simulink model "Solar_Panel_Mathematical_Modelling"  (R2020a)
settings: Solver=VariableStepAuto  StartTime=0.0  StopTime=10.0  RelTol=1e-3
values from neighbouring files (symbols this model uses):
  K = numerator ./ denominator    [Finding_maxima_and_minima_of_any_function.m]    (also in Full_bridge_LLC_resonant_tank_gain_graphs.m; Series_LLC_resonant_converter_calculations.m; Series_LLC_resonant_converter_calculations_2.m; resonant_tank_gain.m)
  Ki = 0.2    [PID_Controller.m]
  n = 1    [Converter_Magnetics_calculations.m]    (also in Series_LLC_resonant_converter_calculations_3.m = 0.0133333333333)
  Ns = 100    [Full_bridge_LLC_resonant_tank_gain_graphs.m]    (also in Series_LLC_resonant_converter_calculations.m; Series_LLC_resonant_converter_calculations_2.m = 75; Series_LLC_resonant_converter_calculations_3.m = 75)
undefined symbols (not defined in the file or in its folder): Eg0, Isc, N, q, Rs, Rsh, Tn, Voc
libraries: simulink x1
settings Model: Creator=HP  LastModifiedBy=HP

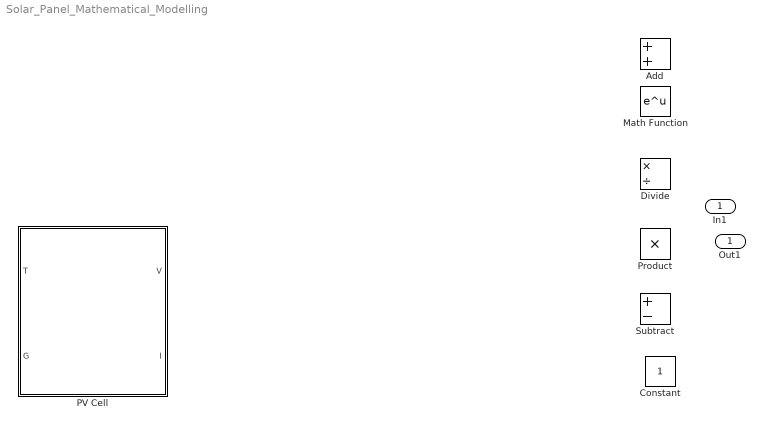
== system Solar_Panel_Mathematical_Modelling ==
  In1 : Inport
  Add : Sum
  Constant : Constant
  Divide : Product  Inputs=*/
  Math Function : Math  SaturateOnIntegerOverflow=on
  PV Cell : Subsystem
  Product : Product
  Subtract : Sum  Inputs=+-
  Out1 : Outport

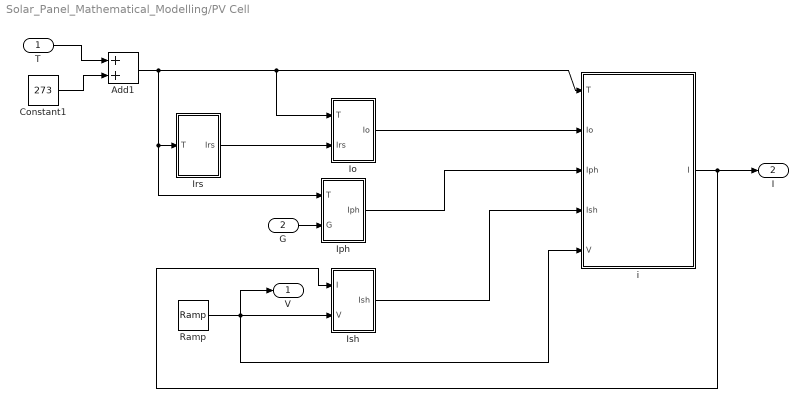
== system Solar_Panel_Mathematical_Modelling/PV Cell ==
  T : Inport
  G : Inport  Port=2
  Add1 : Sum
  Constant1 : Constant  Value=273
  Io : Subsystem
  Iph : Subsystem
  Irs : Subsystem
  Ish : Subsystem
  Ramp : simulink/Sources/Ramp  slope=10  start=0  InitialOutput=0
  i : Subsystem
  V : Outport
  I : Outport  Port=2
  wires:
  Iph/1(Iph) -> i/3(Iph)
  Add1/1 -> Io/1(T), i/1(T), Iph/1(T), Irs/1(T)
  Irs/1(Irs) -> Io/2(Irs)
  T/1 -> Add1/1
  Ish/1(Ish) -> i/4(Ish)
  Constant1/1 -> Add1/2
  i/1(I) -> I/1, Ish/1(I)
  Io/1(Io) -> i/2(Io)
  Ramp/1 -> V/1, Ish/2(V), i/5(V)
  G/1 -> Iph/2(G)

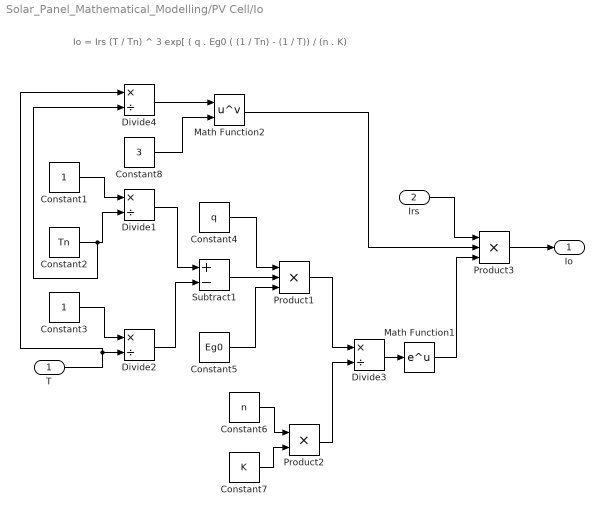
== system Solar_Panel_Mathematical_Modelling/PV Cell/Io ==
  note: Io = Irs (T / Tn) ^ 3 exp[ ( q . Eg0 ( (1 / Tn) - (1 / T)) / (n . K)
  T : Inport
  Irs : Inport  Port=2
  Constant1 : Constant
  Constant2 : Constant  Value=Tn
  Constant3 : Constant
  Constant4 : Constant  Value=q
  Constant5 : Constant  Value=Eg0
  Constant6 : Constant  Value=n
  Constant7 : Constant  Value=K
  Constant8 : Constant  Value=3
  Divide{1..4} (4 alike) : Product  Inputs=*/
  Math Function1 : Math  SaturateOnIntegerOverflow=on
  Math Function2 : Math  Operator=pow  OutputSignalType=real  SaturateOnIntegerOverflow=on
  Product1 : Product  Inputs=3
  Product2 : Product
  Product3 : Product  Inputs=3
  Subtract1 : Sum  Inputs=+-
  Io : Outport
  wires:
  Subtract1/1 -> Product1/2
  T/1 -> Divide2/2, Divide4/1
  Constant7/1 -> Product2/2
  Divide3/1 -> Math Function1/1
  Product3/1 -> Io/1
  Divide4/1 -> Math Function2/1
  Math Function2/1 -> Product3/2
  Constant8/1 -> Math Function2/2
  Constant2/1 -> Divide1/2, Divide4/2
  Product1/1 -> Divide3/1
  Constant1/1 -> Divide1/1
  Divide2/1 -> Subtract1/2
  Irs/1 -> Product3/1
  Constant5/1 -> Product1/3
  Product2/1 -> Divide3/2
  Math Function1/1 -> Product3/3
  Divide1/1 -> Subtract1/1
  Constant4/1 -> Product1/1
  Constant6/1 -> Product2/1
  Constant3/1 -> Divide2/1

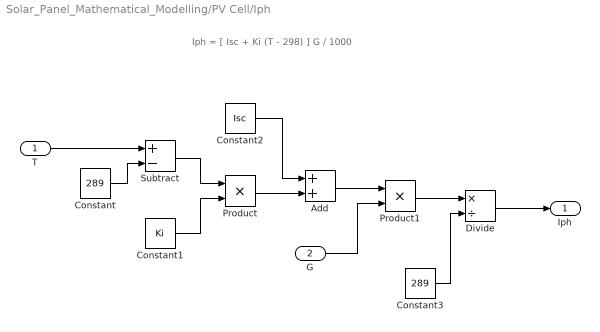
== system Solar_Panel_Mathematical_Modelling/PV Cell/Iph ==
  note: Iph = [ Isc + Ki (T - 298) ] G / 1000
  T : Inport
  G : Inport  Port=2
  Add : Sum
  Constant : Constant  Value=289
  Constant1 : Constant  Value=Ki
  Constant2 : Constant  Value=Isc
  Constant3 : Constant  Value=289
  Divide : Product  Inputs=*/
  Product : Product
  Product1 : Product
  Subtract : Sum  Inputs=+-
  Iph : Outport
  wires:
  Constant3/1 -> Divide/2
  Subtract/1 -> Product/1
  Constant/1 -> Subtract/2
  Constant2/1 -> Add/1
  Product/1 -> Add/2
  T/1 -> Subtract/1
  Constant1/1 -> Product/2
  Product1/1 -> Divide/1
  G/1 -> Product1/2
  Add/1 -> Product1/1
  Divide/1 -> Iph/1

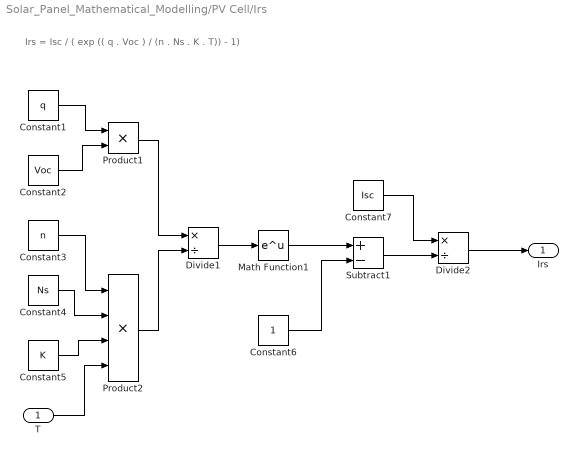
== system Solar_Panel_Mathematical_Modelling/PV Cell/Irs ==
  note: Irs = Isc / ( exp (( q . Voc ) / (n . Ns . K . T)) - 1)
  T : Inport
  Constant1 : Constant  Value=q
  Constant2 : Constant  Value=Voc
  Constant3 : Constant  Value=n
  Constant4 : Constant  Value=Ns
  Constant5 : Constant  Value=K
  Constant6 : Constant
  Constant7 : Constant  Value=Isc
  Divide1 : Product  Inputs=*/
  Divide2 : Product  Inputs=*/
  Math Function1 : Math  SaturateOnIntegerOverflow=on
  Product1 : Product
  Product2 : Product  Inputs=4
  Subtract1 : Sum  Inputs=+-
  Irs : Outport
  wires:
  Constant4/1 -> Product2/2
  Constant5/1 -> Product2/3
  Constant2/1 -> Product1/2
  Product1/1 -> Divide1/1
  Divide2/1 -> Irs/1
  Constant3/1 -> Product2/1
  Product2/1 -> Divide1/2
  Constant1/1 -> Product1/1
  T/1 -> Product2/4
  Constant7/1 -> Divide2/1
  Math Function1/1 -> Subtract1/1
  Subtract1/1 -> Divide2/2
  Constant6/1 -> Subtract1/2
  Divide1/1 -> Math Function1/1

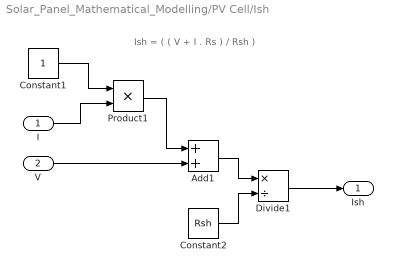
== system Solar_Panel_Mathematical_Modelling/PV Cell/Ish ==
  note: Ish = ( ( V + I . Rs ) / Rsh )
  I : Inport
  V : Inport  Port=2
  Add1 : Sum
  Constant1 : Constant
  Constant2 : Constant  Value=Rsh
  Divide1 : Product  Inputs=*/
  Product1 : Product
  Ish : Outport
  wires:
  I/1 -> Product1/2
  Constant1/1 -> Product1/1
  Add1/1 -> Divide1/1
  V/1 -> Add1/2
  Product1/1 -> Add1/1
  Constant2/1 -> Divide1/2
  Divide1/1 -> Ish/1

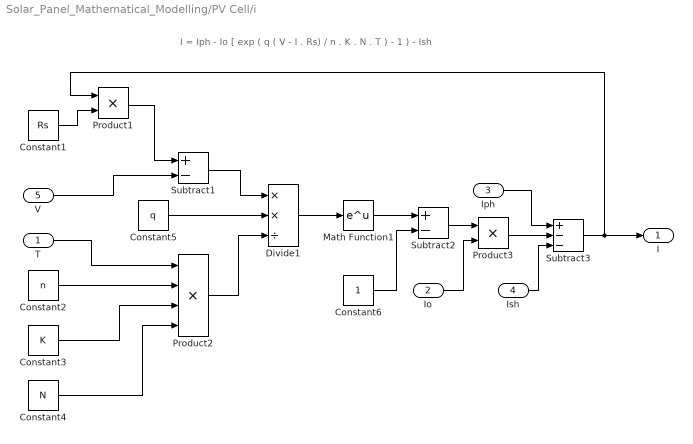
== system Solar_Panel_Mathematical_Modelling/PV Cell/i ==
  note: I = Iph - Io [ exp ( q ( V - I . Rs) / n . K . N . T ) - 1 ) - Ish
  T : Inport
  Io : Inport  Port=2
  Iph : Inport  Port=3
  Ish : Inport  Port=4
  V : Inport  Port=5
  Constant1 : Constant  Value=Rs
  Constant2 : Constant  Value=n
  Constant3 : Constant  Value=K
  Constant4 : Constant  Value=N
  Constant5 : Constant  Value=q
  Constant6 : Constant
  Divide1 : Product  Inputs=**/
  Math Function1 : Math  SaturateOnIntegerOverflow=on
  Product1 : Product
  Product2 : Product  Inputs=4
  Product3 : Product
  Subtract1 : Sum  Inputs=+-
  Subtract2 : Sum  Inputs=+-
  Subtract3 : Sum  Inputs=+--
  I : Outport
  wires:
  Io/1 -> Product3/2
  Math Function1/1 -> Subtract2/1
  Subtract1/1 -> Divide1/1
  Constant2/1 -> Product2/2
  Product2/1 -> Divide1/3
  Constant5/1 -> Divide1/2
  Subtract3/1 -> I/1, Product1/1
  Product3/1 -> Subtract3/2
  Subtract2/1 -> Product3/1
  Constant4/1 -> Product2/4
  Divide1/1 -> Math Function1/1
  Ish/1 -> Subtract3/3
  Product1/1 -> Subtract1/1
  Iph/1 -> Subtract3/1
  T/1 -> Product2/1
  V/1 -> Subtract1/2
  Constant6/1 -> Subtract2/2
  Constant1/1 -> Product1/2
  Constant3/1 -> Product2/3
